simulink model "PI"  (R2020a)
settings: Solver=VariableStepAuto  StartTime=0.0  StopTime=30  RelTol=1e-3
settings Model: Creator=João Fernando Rangel  LastModifiedBy=João Fernando Rangel

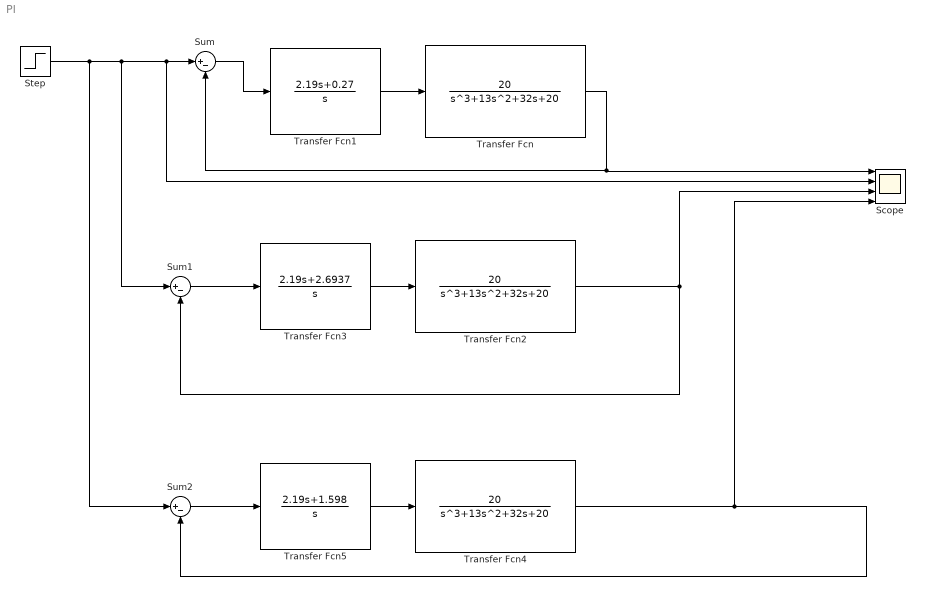
== system PI ==
  Scope : Scope  NumInputPorts=4
  Step : Step  SampleTime=0
  Sum : Sum  Inputs=|+-
  Sum1 : Sum  Inputs=|+-
  Sum2 : Sum  Inputs=|+-
  Transfer Fcn : TransferFcn  Numerator=[0 0 0 20]  Denominator=[1 13 32 20]
  Transfer Fcn1 : TransferFcn  Numerator=[2.19 0.27]  Denominator=[1 0]
  Transfer Fcn2 : TransferFcn  Numerator=[0 0 0 20]  Denominator=[1 13 32 20]
  Transfer Fcn3 : TransferFcn  Numerator=[2.19 2.6937]  Denominator=[1 0]
  Transfer Fcn4 : TransferFcn  Numerator=[0 0 0 20]  Denominator=[1 13 32 20]
  Transfer Fcn5 : TransferFcn  Numerator=[2.19 1.598]  Denominator=[1 0]
  wires:
  Step/1 -> Sum2/1, Scope/2, Sum/1, Sum1/1
  Sum/1 -> Transfer Fcn1/1
  Transfer Fcn1/1 -> Transfer Fcn/1
  Transfer Fcn/1 -> Scope/1, Sum/2
  Sum1/1 -> Transfer Fcn3/1
  Transfer Fcn3/1 -> Transfer Fcn2/1
  Transfer Fcn2/1 -> Scope/3, Sum1/2
  Transfer Fcn5/1 -> Transfer Fcn4/1
  Sum2/1 -> Transfer Fcn5/1
  Transfer Fcn4/1 -> Scope/4, Sum2/2
